simulink model "Sim2"  (R2023b)
settings: Solver=VariableStepAuto  StartTime=0.0  StopTime=10  RelTol=1e-3
model workspace (MAT data in the model file):
  b = 10
  g = 9.8
  l = 0.8
  m = 2
settings Model: Creator=surrlim  LastModifiedBy=surrlim

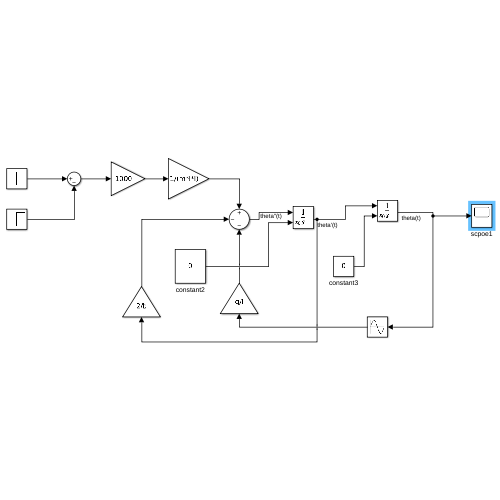
[thumbnail: Simulink's stored preview of the top-level diagram]
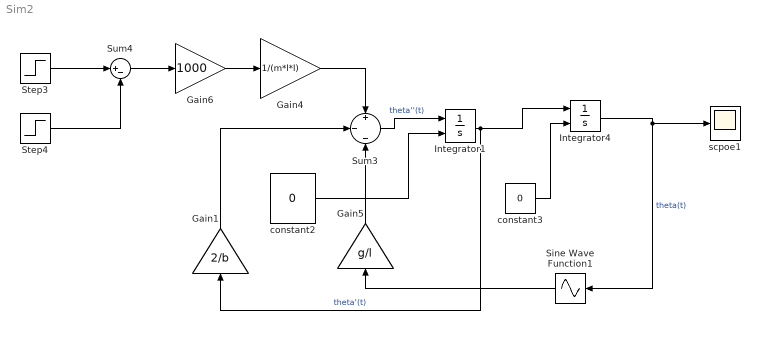
== system Sim2 ==
  Gain1 : Gain  Gain=2/b
  Gain4 : Gain  Gain=1/(m*l*l)
  Gain5 : Gain  Gain=g/l
  Gain6 : Gain  Gain=1000
  Integrator1 : Integrator  InitialConditionSource=external  InitialCondition=1/(m*l*l)
  Integrator4 : Integrator  InitialConditionSource=external
  Sine Wave Function1 : Sin  TimeSource=Use external signal  Frequency=1/(2*pi)  SampleTime=0
  Step3 : Step  Time=0  SampleTime=0
  Step4 : Step  Time=0.001  SampleTime=0
  Sum3 : Sum  Inputs=+|-|-
  Sum4 : Sum  Inputs=|+-
  constant2 : Constant  Value=0
  constant3 : Constant  Value=0
  scpoe1 : Scope
  wires:
  Integrator4/1 -> Sine Wave Function1/1, scpoe1/1  "theta(t)"
  Sine Wave Function1/1 -> Gain5/1
  Gain5/1 -> Sum3/3
  constant3/1 -> Integrator4/2
  Step4/1 -> Sum4/2
  Integrator1/1 -> Gain1/1, Integrator4/1  "theta'(t)"
  Sum3/1 -> Integrator1/1  "theta''(t)"
  Gain4/1 -> Sum3/1
  Step3/1 -> Sum4/1
  constant2/1 -> Integrator1/2
  Sum4/1 -> Gain6/1
  Gain6/1 -> Gain4/1
  Gain1/1 -> Sum3/2
